simulink model "hw4_1d_helicopter"  (R2014a)
settings: Solver=ode45  StartTime=0.0  StopTime=0.2  RelTol=1e-3
model workspace (MAT data in the model file):
  a = 5
  T_top = 4
  Kp = 30
  Ki = 12000
settings Model: Creator=feisele  LastModifiedBy=feisele
settings DebuggingCC: SolverPrmCheckMsg=none

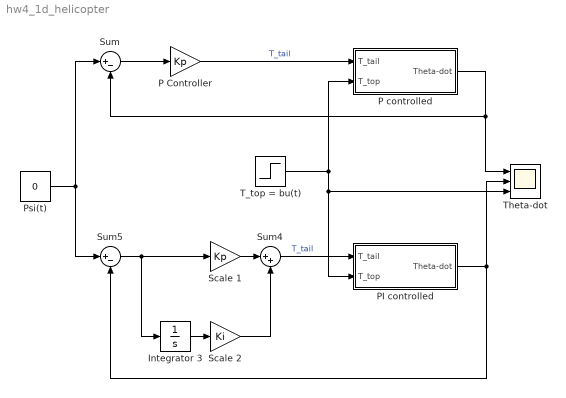
== system hw4_1d_helicopter ==
  Integrator 3 : Integrator
  P Controller : Gain  Gain=Kp
  P controlled : Subsystem
  PI controlled : Subsystem
  Psi(t) : Constant  Value=0
  Scale 1 : Gain  Gain=Kp
  Scale 2 : Gain  Gain=Ki
  Sum : Sum  Inputs=|+-
  Sum4 : Sum  Inputs=|++
  Sum5 : Sum  Inputs=|+-
  T_top = bu(t) : Step  Time=0.1  After=T_top  SampleTime=0
  Theta-dot : Scope  NumInputPorts=3
      settings: ShowLegends=on  YMin=-0.2~-0.2~-5  YMax=0.2~0.2~5
  wires:
  Psi(t)/1 -> Sum5/1, Sum/1
  Sum/1 -> P Controller/1
  P Controller/1 -> P controlled/1(T_tail)  "T_tail"
  P controlled/1(Theta-dot) -> Sum/2, Theta-dot/1
  Sum5/1 -> Integrator 3/1, Scale 1/1
  Integrator 3/1 -> Scale 2/1
  Scale 2/1 -> Sum4/2
  Scale 1/1 -> Sum4/1
  Sum4/1 -> PI controlled/1(T_tail)  "T_tail"
  PI controlled/1(Theta-dot) -> Theta-dot/2, Sum5/2
  T_top = bu(t)/1 -> P controlled/2(T_top), PI controlled/2(T_top), Theta-dot/3

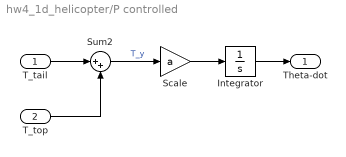
== system hw4_1d_helicopter/P controlled ==
  T_tail : Inport
  T_top : Inport  Port=2
  Integrator : Integrator
  Scale : Gain  Gain=a
  Sum2 : Sum  Inputs=|++
  Theta-dot : Outport
  wires:
  T_tail/1 -> Sum2/1
  T_top/1 -> Sum2/2
  Integrator/1 -> Theta-dot/1
  Sum2/1 -> Scale/1  "T_y"
  Scale/1 -> Integrator/1

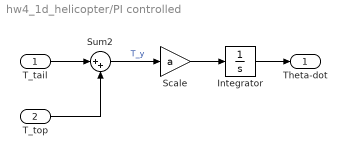
== system hw4_1d_helicopter/PI controlled ==
  T_tail : Inport
  T_top : Inport  Port=2
  Integrator : Integrator
  Scale : Gain  Gain=a
  Sum2 : Sum  Inputs=|++
  Theta-dot : Outport
  wires:
  T_tail/1 -> Sum2/1
  T_top/1 -> Sum2/2
  Integrator/1 -> Theta-dot/1
  Sum2/1 -> Scale/1  "T_y"
  Scale/1 -> Integrator/1
